simulink model "watertank_STL_test_breach"  (R2018b)
settings: Solver=FixedStepAuto  StartTime=0.0  StopTime=tspan(end)  FixedStep=0.01  RelTol=1e-3
model workspace (MAT data in the model file):
  A = 20
  a = 2
  b = 5
libraries: neural x66, simulink x3
(part 3 of 3)

== system watertank_STL_test_breach/NN/Layer 3/Delays 1 ==
  "p{3}" : Inport  PortDimensions=30
      mask Display: e = 0.06;c1 = [120 230 180]/255;c2 = ([120 230 180]+0)/(256+128);c3 = ([120 230 180]+128)/(256+128);patch([0 1 1 0],[0 0 1 1],c1);patch([0 1 1 1-e 1-e 0+e],[0 0 1 1-e 0+e 0+e],c2);patch([0 0 1 1-e 0+e 0+e],[0 1 1 1-e 1-e 0+e],c3);plot([0 1 1 0 0],[0 0 1 1 0]);
  mux : Mux  Inputs=1
      mask Display: e = 0.06;c1 = [120 150 230]/255;c2 = ([120 150 230]+0)/383;c3 = ([120 150 230]+128)/383;patch([0 1 1 0],[0 0 1 1],c1);patch([0 1 1 1-e 1-e 0+e],[0 0 1 1-e 0+e 0+e],c2);patch([0 0 1 1-e 0+e 0+e],[0 1 1 1-e 1-e 0+e],c3);plot([0 1 1 0 0],[0 0 1 1 0]);disp('Mux')
  "pd{3,2}" : Outport
      mask Display: e = 0.06;c1 = [120 230 180]/255;c2 = ([120 230 180]+0)/(256+128);c3 = ([120 230 180]+128)/(256+128);patch([0 1 1 0],[0 0 1 1],c1);patch([0 1 1 1-e 1-e 0+e],[0 0 1 1-e 0+e 0+e],c2);patch([0 0 1 1-e 0+e 0+e],[0 1 1 1-e 1-e 0+e],c3);plot([0 1 1 0 0],[0 0 1 1 0]);
  wires:
  "p{3}"/1 -> mux/1
  mux/1 -> "pd{3,2}"/1

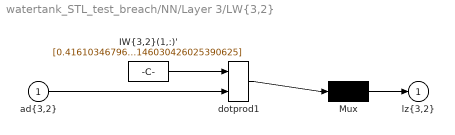
== system watertank_STL_test_breach/NN/Layer 3/LW{3,2} ==
  "ad{3,2}" : Inport  PortDimensions=30
      mask Display: e = 0.06;c1 = [120 230 180]/255;c2 = ([120 230 180]+0)/(256+128);c3 = ([120 230 180]+128)/(256+128);patch([0 1 1 0],[0 0 1 1],c1);patch([0 1 1 1-e 1-e 0+e],[0 0 1 1-e 0+e 0+e],c2);patch([0 0 1 1-e 0+e 0+e],[0 1 1 1-e 1-e 0+e],c3);plot([0 1 1 0 0],[0 0 1 1 0]);
  "IW{3,2}(1,:)'" : Constant  Value=[0.416103467969001494797254281365894712507724761962890625;1.045850379342733393883690951042808592319488525390625;0.335157921609311737487502114163362421095371246337890625;-0.63209023314226786549596681652474217116832733154296875;0.259083830730509501183433940241229720413684844970703125;0.84720733388366642468980671765166334807872772216796875;-0.7034163063867711063181786812492646276950836181640625;-0.81217489601318215708403158714645542204380035400390625;-0.023579935386392116003495544873658218421041965484619140625;0.14362150743602841718171703178086318075656890869140625;-0.74595902682359682689394730914500541985034942626953125;-0.7032528594690699019764679178479127585887908935546875;0.673250279104056659207344637252390384674072265625;0.685338817766062202707644246402196586132049560546875;0.642296500032360828669197871931828558444976806640625;-0.5850669548917706297430640915990807116031646728515625;0.582388997868080959818826158880256116390228271484375;0.2506278300594739771867125455173663794994354248046875;-0.00975883965735367155114321491282680653966963291168212890625;0.048009532608977945056238922916236333549022674560546875;-0.7143236005786428588493208735599182546138763427734375;0.51241008146831779068719470160431228578090667724609375;0.01477649819101171761726032372052941354922950267791748046875;-0.466282828659459747111526439766748808324337005615234375;-0.57499417653282858253760423394851386547088623046875;-0.837478494095236225547296271543018519878387451171875;0.824297084785498679337933936039917171001434326171875;-0.89095764587085357621987213860847987234592437744140625;-0.297390812580489993788290803422569297254085540771484375;0.2206744948577538389944407981602125801146030426025390625]
      mask Display: e = 0.06;c1 = [120 150 230]/255;c2 = ([120 150 230]+0)/383;c3 = ([120 150 230]+128)/383;patch([0 1 1 0],[0 0 1 1],c1);patch([0 1 1 1-e 1-e 0+e],[0 0 1 1-e 0+e 0+e],c2);patch([0 0 1 1-e 0+e 0+e],[0 1 1 1-e 1-e 0+e],c3);plot([0 1 1 0 0],[0 0 1 1 0]);disp('weights');
  Mux : Mux  Inputs=1
      mask Display: e = 0.06;c1 = [120 150 230]/255;c2 = ([120 150 230]+0)/383;c3 = ([120 150 230]+128)/383;patch([0 1 1 0],[0 0 1 1],c1);patch([0 1 1 1-e 1-e 0+e],[0 0 1 1-e 0+e 0+e],c2);patch([0 0 1 1-e 0+e 0+e],[0 1 1 1-e 1-e 0+e],c3);plot([0 1 1 0 0],[0 0 1 1 0]);disp('Mux');
  dotprod1 : neural/Weight Functions/dotprod
  "lz{3,2}" : Outport
      mask Display: e = 0.06;c1 = [120 230 180]/255;c2 = ([120 230 180]+0)/(256+128);c3 = ([120 230 180]+128)/(256+128);patch([0 1 1 0],[0 0 1 1],c1);patch([0 1 1 1-e 1-e 0+e],[0 0 1 1-e 0+e 0+e],c2);patch([0 0 1 1-e 0+e 0+e],[0 1 1 1-e 1-e 0+e],c3);plot([0 1 1 0 0],[0 0 1 1 0]);
  wires:
  "IW{3,2}(1,:)'"/1 -> dotprod1/1
  "ad{3,2}"/1 -> dotprod1/2
  dotprod1/1 -> Mux/1
  Mux/1 -> "lz{3,2}"/1
